simulink model "Vehicle_Dynamic_Simulator"  (R2021b)
settings: Solver=VariableStepAuto  StartTime=0.0  StopTime=200  RelTol=1e-3
undefined symbols (not defined in the file): Path
libraries: Solver_SF x2, mpclib x1, sldrtlib x1
(part 1 of 2)
settings Model: Creator=li.ang  LastModifiedBy=li.ang
settings SFSimCC: SimTargetLang=C++
settings ConfigComp: PLC_TargetIDE=codesys23  PLC_MultiTBSigbuilderTimeRange=off  PLC_InlineEnumCastFunction=off

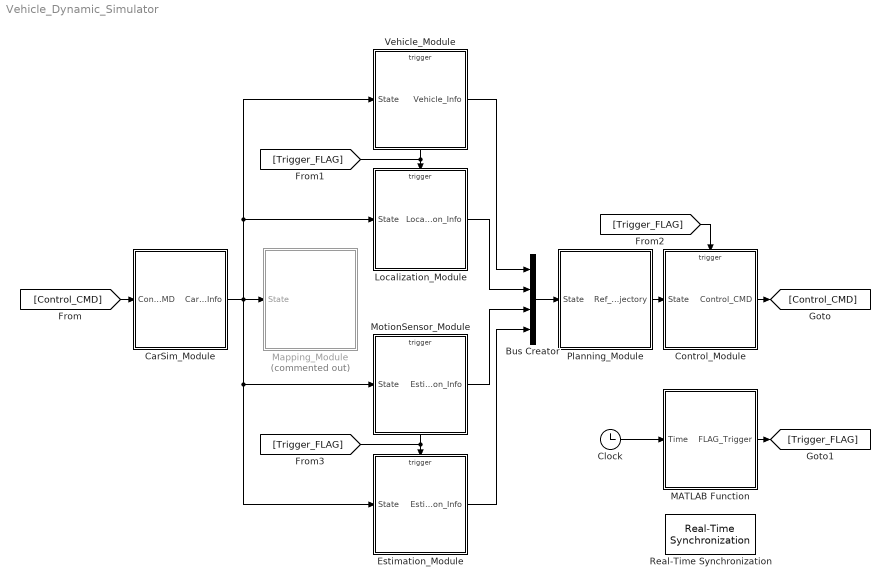
== system Vehicle_Dynamic_Simulator ==
  Bus Creator : BusCreator  Inputs=4
  CarSim_Module : Subsystem  mask{LonFlag=on, LatFlag=on}
      mask prompts: LonFlag "use custom lon controller"; LatFlag "use custom lat controller"
      mask Display: image('TruckSim.png'); % 使用工具条上的 "编辑图像" 进行更改。
  Clock : Clock
  Control_Module : Subsystem
  Estimation_Module : Subsystem  mask{VehicleFlag=Truck_106_Daimler_Auman, ModelFlag=Static 2DOF Vehicle Model}
      mask prompts: VehicleFlag "Select Test Vehicle"; ModelFlag "Model Type"
      mask TypeOptions VehicleFlag: Truck_106_Daimler_Auman
      mask TypeOptions ModelFlag: Static 2DOF Vehicle Model | Static 2DOF Error Model | Dynamic 2DOF Vehicle Model | Dynamic 2DOF Error Model
      mask Display: addpath('Pictures');
  Localization_Module : Subsystem  mask{FLAGS_choose_path=Test: Step Curvature Response: 10m Radius, FLAGS_enable_preview=on, FLAGS_preview_window=0}
      mask prompts: FLAGS_choose_path "Select Path"; FLAGS_enable_preview "Enable Preview"; FLAGS_preview_window "Input Preview Window"
      mask init:
      | % Add Search Path
      | addpath('Scenarios');
      | addpath('Scenarios\Scenario_Test_Flat_Pad');
      | 
      | % Test Road Selector
      | switch FLAGS_choose_path
      |     case 1
      |         load('Path_Curvature_Step_Response_8m_Radius.mat');
      |     case 2
      |         load('Path_Curvature_Step_Response_10m_Radius.mat');
      |     case 3
      |         load('Path_Curvature_Step_Response_16m_Radius.mat');
      |     case 4
      |         load('Path_Curvature_Step_Response_20m_Radius.mat');
      |     case 5
      |         load('Path_Curvature_Step_Response_40m_Radius.mat');
      |     case 6
      |         load('Path_Curvature_Step_Response_50m_Radius.mat');
      |     case 7
      |         load('Path_Curvature_Step_Response_80m_Radius.mat');
      |     case 8
      |         load('Path_Curvature_Step_Response_100m_Radius.mat');
      | 
      | %     case 2
      | %         load('MCity_M_Loop.mat')
      | % 
      | %     case 3      % Road: Course2D
      | %         load('Path_HandlingCourse.mat');
      | % 
      | %     case 8      % Road: Course3D
      | %         Path = load('Course3D.mat');
      | %         Index      = Path.Road.Index
      | %         Station    = Path.Road.S;
      | %         X_Global   = Path.Road.X;
      | %         Y_Global   = Path.Road.Y;
      | %         Theta      = Path.Road.Theta;
      | %         Kappa      = Path.Road.Kappa; 
      |         
      | %     case 1      % Step Curvature: Kappa = 0.01
      | %         Centerline = load('Step_Kappa_0.01.mat');
      | %         Index      = Centerline.Road.Index
      | %         Station    = Centerline.Road.S;
      | %         X_Global   = Centerline.Road.X;
      | %         Y_Global   = Centerline.Road.Y;
      | %         Theta      = Centerline.Road.Theta;
      | %         Kappa      = Centerline.Road.Kappa;
      | %     case 2      % Step Curvature: Kappa = 0.02
      | %         Centerline = load('Step_Kappa_0.02.mat');
      | %         Index      = Centerline.Road.Index
      | %         Station    = Centerline.Road.S;
      | %         X_Global   = Centerline.Road.X;
      | %         Y_Global   = Centerline.Road.Y;
      | %         Theta      = Centerline.Road.Theta;
      | %         Kappa      = Centerline.Road.Kappa;  
      | %     case 3      % Step Curvature: Kappa = 0.05
      | %         Centerline = load('Step_Kappa_0.05.mat');
      | %         Index      = Centerline.Road.Index
      | %         Station    = Centerline.Road.S;
      | %         X_Global   = Centerline.Road.X;
      | %         Y_Global   = Centerline.Road.Y;
      | %         Theta      = Centerline.Road.Theta;
      | %         Kappa      = Centerline.Road.Kappa;
      | %     case 4      % Ramp Curvature: dKappa = 0.01
      | %         Centerline = load('Ramp_dKappa_0.01.mat');
      | %         Index      = Centerline.Road.Index
      | %         Station    = Centerline.Road.S;
      | %         X_Global   = Centerline.Road.X;
      | %         Y_Global   = Centerline.Road.Y;
      | %         Theta      = Centerline.Road.Theta;
      | %         Kappa      = Centerline.Road.Kappa;
      | %     case 5      % Road: uTurn
      | %         Centerline = load('uTurn.mat');
      | %         Index      = Centerline.Road.Index
      | %         Station    = Centerline.Road.S;
      | %         X_Global   = Centerline.Road.X;
      | %         Y_Global   = Centerline.Road.Y;
      | %         Theta      = Centerline.Road.Theta;
      | %         Kappa      = Centerline.Road.Kappa;
      | %     case 6      % Road: Highway
      | %         Centerline = load('Highway.mat');
      | %         Index      = Centerline.Road.Index
      | %         Station    = Centerline.Road.S;
      | %         X_Global   = Centerline.Road.X;
      | %         Y_Global   = Centerline.Road.Y;
      | %         Theta      = Centerline.Road.Theta;
      | %         Kappa      = Centerline.Road.Kappa;
      | end
      mask TypeOptions FLAGS_choose_path: Test: Step Curvature Response: 8m Radius | Test: Step Curvature Response: 10m Radius | Test: Step Curvature Response: 16m Radius | Test: Step Curvature Response: 20m Radius | Test: Step Curvature Response: 40m Radius | Test: Step Curvature Response: 50m Radius | Test: Step Curvature Response: 80m Radius | Test: Step Curvature Response: 100m Radius
      mask Display:
      | addpath('Pictures');
      | image('Road.png');
  MATLAB Function : MATLAB Function  TreatAsAtomicUnit=on
  Mapping_Module : Subsystem  Commented=on
  MotionSensor_Module : Subsystem  mask{VehicleFlag=Truck_106_Daimler_Auman, ModelFlag=Static 2DOF Vehicle Model}
      mask prompts: VehicleFlag "Select Test Vehicle"; ModelFlag "Model Type"
      mask TypeOptions VehicleFlag: Truck_106_Daimler_Auman
      mask TypeOptions ModelFlag: Static 2DOF Vehicle Model | Static 2DOF Error Model | Dynamic 2DOF Vehicle Model | Dynamic 2DOF Error Model
      mask Display: addpath('Pictures');
  Planning_Module : Subsystem
  Real-Time Synchronization : sldrtlib/Real-Time Synchronization  SampleTime=0.1  MaxMissedTicks=10  ShowMissedTicks=off  YieldWhenWaiting=off
  Vehicle_Module : Subsystem  mask{VehicleFlag=Truck_106_Daimler_Auman, ModelFlag=Static 2DOF Vehicle Model}
      mask prompts: VehicleFlag "Select Test Vehicle"; ModelFlag "Model Type"
      mask init:
      | % Add Search Path
      | addpath('Vehicles');
      | 
      | % Test Vehicle Selector
      | % switch VehicleFlag
      | %     case 1
      | %         Vehicle         = load('Truck_106_Daimler_Auman.mat').Vehicle;
      | %         TotalMass       = Vehicle.TotalMass;
      | %         TotalInertia    = Vehicle.TotalInertia;
      | %         TyreStiffness   = Vehicle.AxleStiffness;
      | %         AxlePosition    = Vehicle.AxlePosition;
      | %     case 2
      | %     case 3
      | %     case 4
      | %         Vehicle         = load('Truck_106_Daimler_Auman.mat').Vehicle;
      | %         TotalMass       = Vehicle.TotalMass;
      | %         TotalInertia    = Vehicle.TotalInertia;
      | %         TyreStiffness   = Vehicle.AxleStiffness;
      | %         AxlePosition    = Vehicle.AxlePosition;
      | %         ...
      | % end
      mask TypeOptions VehicleFlag: Truck_106_Daimler_Auman
      mask TypeOptions ModelFlag: Static 2DOF Vehicle Model | Static 2DOF Error Model | Dynamic 2DOF Vehicle Model | Dynamic 2DOF Error Model
      mask Display:
      | addpath('Pictures');
      | image('Vehicle_Module.png');
  wires:
  CarSim_Module/1(CarSim_Info) -> Mapping_Module/1(State), Estimation_Module/1(State), MotionSensor_Module/1(State), Vehicle_Module/1(State), Localization_Module/1(State)
  Control_Module/1(Control_CMD) -> [Control_CMD]
  Bus Creator/1 -> Planning_Module/1(State)
  Planning_Module/1(Ref_Trajectory) -> Control_Module/1(State)
  MATLAB Function/1(FLAG_Trigger) -> [Trigger_FLAG]
  Clock/1 -> MATLAB Function/1(Time)
  [Trigger_FLAG] -> Localization_Module/Trigger, Vehicle_Module/Trigger
  [Trigger_FLAG] -> Control_Module/Trigger
  [Trigger_FLAG] -> Estimation_Module/Trigger, MotionSensor_Module/Trigger
  [Control_CMD] -> CarSim_Module/1(Control_CMD)
  Vehicle_Module/1(Vehicle_Info) -> Bus Creator/1
  Localization_Module/1(Localization_Info) -> Bus Creator/2
  MotionSensor_Module/1(Estimation_Info) -> Bus Creator/3
  Estimation_Module/1(Estimation_Info) -> Bus Creator/4

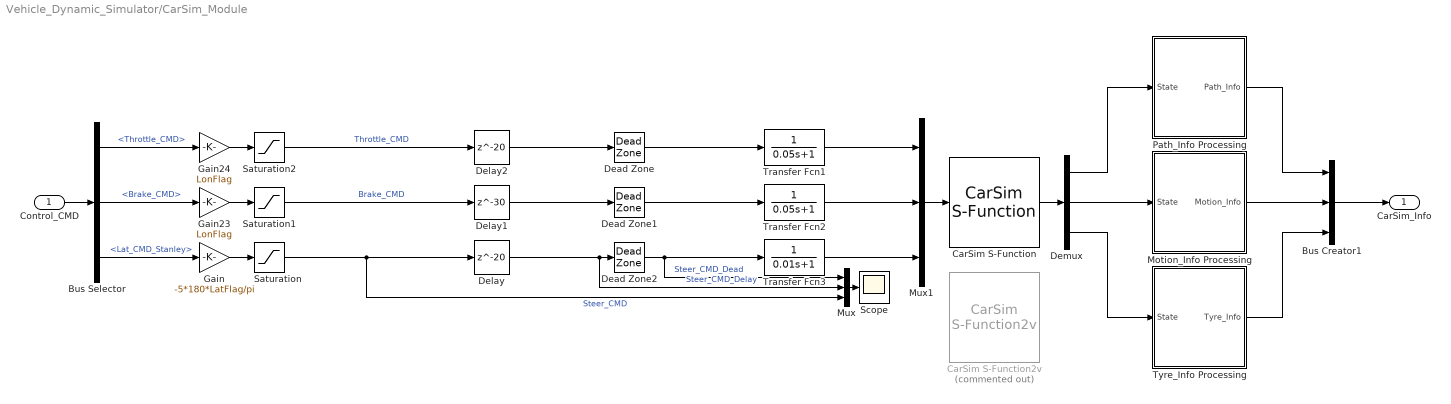
== system Vehicle_Dynamic_Simulator/CarSim_Module ==
  Control_CMD : Inport
  Bus Creator1 : BusCreator  Inputs=3
  Bus Selector : BusSelector  OutputSignals=Lon_CMD.Throttle_CMD,Lon_CMD.Brake_CMD,Lat_CMD.Lat_CMD_Stanley
  CarSim S-Function : Solver_SF/CarSim S-Function  Priority=1  SIMFILE=simfile.sim
  CarSim S-Function2v : Solver_SF/CarSim S-Function2v  Priority=1  Commented=on  SIMFILE=CarSimfile.sim
      settings: SourceProductName=CarSim S-Function
  Dead Zone : DeadZone  LowerValue=0  UpperValue=0.05  SaturateOnIntegerOverflow=on
  Dead Zone1 : DeadZone  LowerValue=0  UpperValue=0.05  SaturateOnIntegerOverflow=on
  Dead Zone2 : DeadZone  LowerValue=-1  UpperValue=1  SaturateOnIntegerOverflow=on
  Delay : Delay  DelayLength=20
  Delay1 : Delay  DelayLength=30  SampleTime=0.01
  Delay2 : Delay  DelayLength=20  SampleTime=0.01
  Demux : Demux  Outputs=[14, 20, 44]
  Gain : Gain  Gain=-5*180*LatFlag/pi
  Gain23 : Gain  Gain=LonFlag
  Gain24 : Gain  Gain=LonFlag
  Motion_Info Processing : Subsystem
  Mux : Mux  Inputs=3
  Mux1 : Mux  Inputs=3
  Path_Info Processing : Subsystem
  Saturation : Saturate  UpperLimit=+540  LowerLimit=-540
  Saturation1 : Saturate  UpperLimit=+1000  LowerLimit=-1000
  Saturation2 : Saturate  UpperLimit=+1000  LowerLimit=-1000
  Scope : Scope
  Transfer Fcn1 : TransferFcn  Denominator=[0.05 1]
  Transfer Fcn2 : TransferFcn  Denominator=[0.05 1]
  Transfer Fcn3 : TransferFcn  Denominator=[0.01 1]
  Tyre_Info Processing : Subsystem
  CarSim_Info : Outport
  wires:
  Bus Creator1/1 -> CarSim_Info/1
  Mux1/1 -> CarSim S-Function/1
  Demux/1 -> Path_Info Processing/1(State)
  CarSim S-Function/1 -> Demux/1
  Demux/2 -> Motion_Info Processing/1(State)
  Demux/3 -> Tyre_Info Processing/1(State)
  Motion_Info Processing/1(Motion_Info) -> Bus Creator1/2
  Path_Info Processing/1(Path_Info) -> Bus Creator1/1
  Tyre_Info Processing/1(Tyre_Info) -> Bus Creator1/3
  Saturation/1 -> Mux/3, Delay/1  "Steer_CMD"
  Dead Zone/1 -> Transfer Fcn1/1
  Mux/1 -> Scope/1
  Dead Zone1/1 -> Transfer Fcn2/1
  Delay/1 -> Mux/2, Dead Zone2/1  "Steer_CMD_Delay"
  Gain23/1 -> Saturation1/1
  Control_CMD/1 -> Bus Selector/1
  Delay2/1 -> Dead Zone/1
  Gain24/1 -> Saturation2/1
  Saturation2/1 -> Delay2/1  "Throttle_CMD"
  Dead Zone2/1 -> Mux/1, Transfer Fcn3/1  "Steer_CMD_Dead"
  Delay1/1 -> Dead Zone1/1
  Saturation1/1 -> Delay1/1  "Brake_CMD"
  Gain/1 -> Saturation/1
  Bus Selector/1 -> Gain24/1  "<Throttle_CMD>"
  Bus Selector/2 -> Gain23/1  "<Brake_CMD>"
  Bus Selector/3 -> Gain/1  "<Lat_CMD_Stanley>"
  Transfer Fcn2/1 -> Mux1/2
  Transfer Fcn1/1 -> Mux1/1
  Transfer Fcn3/1 -> Mux1/3

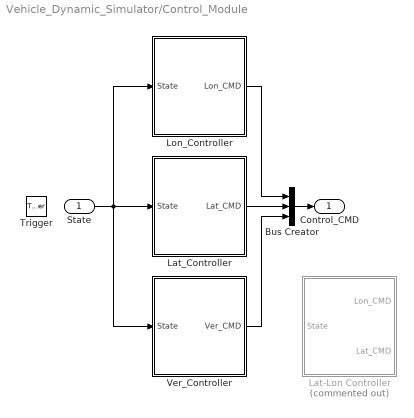
== system Vehicle_Dynamic_Simulator/Control_Module ==
  State : Inport
  Trigger : TriggerPort  VariantControl=(inherit)  PortDimensions=1
  Bus Creator : BusCreator  Inputs=3
  Lat-Lon Controller : Subsystem  Commented=on
  Lat_Controller : Subsystem
  Lon_Controller : Subsystem
  Ver_Controller : Subsystem
  Control_CMD : Outport
  wires:
  Bus Creator/1 -> Control_CMD/1
  Lon_Controller/1(Lon_CMD) -> Bus Creator/1
  State/1 -> Ver_Controller/1(State), Lat_Controller/1(State), Lon_Controller/1(State)
  Lat_Controller/1(Lat_CMD) -> Bus Creator/2
  Ver_Controller/1(Ver_CMD) -> Bus Creator/3

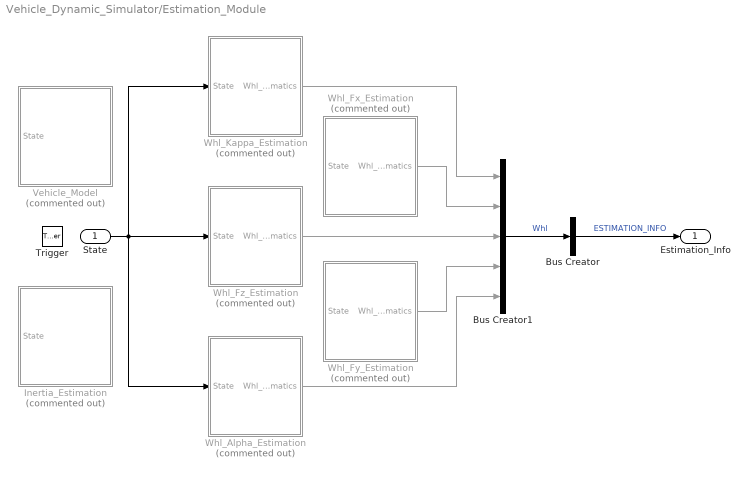
== system Vehicle_Dynamic_Simulator/Estimation_Module ==
  State : Inport
  Trigger : TriggerPort  VariantControl=(inherit)  PortDimensions=1
  Bus Creator : BusCreator  Inputs=1
  Bus Creator1 : BusCreator  Inputs=5
  Inertia_Estimation : Subsystem  Commented=on
  Vehicle_Model : Subsystem  Commented=on
  Whl_Alpha_Estimation : Subsystem  Commented=on
  Whl_Fx_Estimation : Subsystem  Commented=on
  Whl_Fy_Estimation : Subsystem  Commented=on
  Whl_Fz_Estimation : Subsystem  Commented=on
  Whl_Kappa_Estimation : Subsystem  Commented=on
  Estimation_Info : Outport
  wires:
  State/1 -> Whl_Fz_Estimation/1(State), Whl_Alpha_Estimation/1(State), Whl_Kappa_Estimation/1(State)
  Bus Creator/1 -> Estimation_Info/1  "ESTIMATION_INFO"
  Whl_Kappa_Estimation/1(Whl_Kinematics) -> Bus Creator1/1
  Bus Creator1/1 -> Bus Creator/1  "Whl"
  Whl_Fz_Estimation/1(Whl_Kinematics) -> Bus Creator1/3
  Whl_Fx_Estimation/1(Whl_Kinematics) -> Bus Creator1/2
  Whl_Fy_Estimation/1(Whl_Kinematics) -> Bus Creator1/4
  Whl_Alpha_Estimation/1(Whl_Kinematics) -> Bus Creator1/5

== system Vehicle_Dynamic_Simulator/Localization_Module ==
  State : Inport
  Trigger : TriggerPort  VariantControl=(inherit)  PortDimensions=1
  Bus Creator : BusCreator  Inputs=3
  Error_Calculation : Subsystem
  Geo_Calculation : Subsystem
  Prev_Calculation : Subsystem
  Localization_Info : Outport
  wires:
  State/1 -> Geo_Calculation/1(State), Prev_Calculation/1(State), Error_Calculation/1(State)
  Bus Creator/1 -> Localization_Info/1  "LOCALIZATION_INFO"
  Error_Calculation/1(Path_Error_Info) -> Bus Creator/1
  Prev_Calculation/1(Path_Prev_Info) -> Bus Creator/3
  Geo_Calculation/1(Path_Error_Info) -> Bus Creator/2

== system Vehicle_Dynamic_Simulator/Mapping_Module ==
  State : Inport
  Bus Selector : BusSelector  OutputSignals=PATH_INFO.Path_S_Ref,PATH_INFO.Path_X_Ref,PATH_INFO.Path_Y_Ref,PATH_INFO.Path_Kappa_Ref
  Scope : Scope  NumInputPorts=4
  To Workspace : ToWorkspace  VariableName=S  SaveFormat=Timeseries  SampleTime=0.02
  To Workspace1 : ToWorkspace  VariableName=X  SaveFormat=Timeseries  SampleTime=0.02
  To Workspace2 : ToWorkspace  VariableName=Y  SaveFormat=Timeseries  SampleTime=0.02
  To Workspace3 : ToWorkspace  VariableName=Kappa  SaveFormat=Timeseries  SampleTime=0.02
  wires:
  State/1 -> Bus Selector/1
  Bus Selector/1 -> To Workspace/1, Scope/1  "<Path_S_Ref>"
  Bus Selector/2 -> To Workspace1/1, Scope/2  "<Path_X_Ref>"
  Bus Selector/3 -> To Workspace2/1, Scope/3  "<Path_Y_Ref>"
  Bus Selector/4 -> Scope/4, To Workspace3/1  "<Path_Kappa_Ref>"

== system Vehicle_Dynamic_Simulator/MotionSensor_Module ==
  State : Inport
  Trigger : TriggerPort  VariantControl=(inherit)  PortDimensions=1
  Bus Selector : BusSelector  OutputSignals=MOTION_INFO
  Estimation_Info : Outport
  wires:
  Bus Selector/1 -> Estimation_Info/1  "<MOTION_INFO>"
  State/1 -> Bus Selector/1

== system Vehicle_Dynamic_Simulator/Planning_Module ==
  State : Inport
  Ref_Trajectory : Outport
  wires:
  State/1 -> Ref_Trajectory/1

== system Vehicle_Dynamic_Simulator/Vehicle_Module ==
  State : Inport
  Trigger : TriggerPort  VariantControl=(inherit)  PortDimensions=1
  Vehicle_Info : Outport
  wires:
  State/1 -> Vehicle_Info/1  "VEHICLE_INFO"

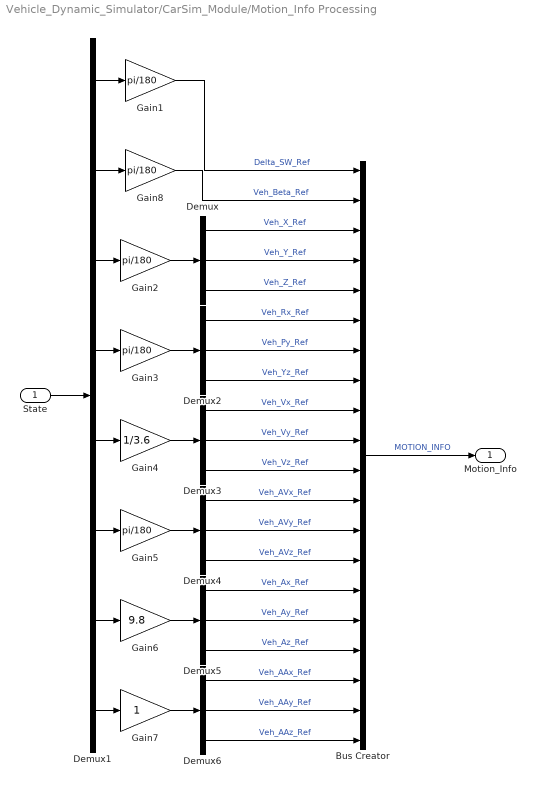
== system Vehicle_Dynamic_Simulator/CarSim_Module/Motion_Info Processing ==
  State : Inport
  Bus Creator : BusCreator  Inputs=20
  Demux{,2..6} (6 alike) : Demux  Outputs=3
  Demux1 : Demux  Outputs=[1, 1, 3, 3, 3, 3, 3, 3]
  Gain{1..3,5,8} (5 alike) : Gain  Gain=pi/180
  Gain4 : Gain  Gain=1/3.6
  Gain6 : Gain  Gain=9.8
  Gain7 : Gain
  Motion_Info : Outport
  wires:
  State/1 -> Demux1/1
  Bus Creator/1 -> Motion_Info/1  "MOTION_INFO"
  Demux1/1 -> Gain1/1
  Gain1/1 -> Bus Creator/1  "Delta_SW_Ref"
  Demux1/6 -> Gain5/1
  Demux5/1 -> Bus Creator/15  "Veh_Ax_Ref"
  Demux4/1 -> Bus Creator/12  "Veh_AVx_Ref"
  Demux1/5 -> Gain4/1
  Demux5/2 -> Bus Creator/16  "Veh_Ay_Ref"
  Demux4/2 -> Bus Creator/13  "Veh_AVy_Ref"
  Demux3/2 -> Bus Creator/10  "Veh_Vy_Ref"
  Demux3/3 -> Bus Creator/11  "Veh_Vz_Ref"
  Gain7/1 -> Demux6/1
  Demux1/8 -> Gain7/1
  Demux4/3 -> Bus Creator/14  "Veh_AVz_Ref"
  Demux6/2 -> Bus Creator/19  "Veh_AAy_Ref"
  Demux1/7 -> Gain6/1
  Demux6/1 -> Bus Creator/18  "Veh_AAx_Ref"
  Gain5/1 -> Demux4/1
  Demux5/3 -> Bus Creator/17  "Veh_Az_Ref"
  Demux3/1 -> Bus Creator/9  "Veh_Vx_Ref"
  Gain4/1 -> Demux3/1
  Gain6/1 -> Demux5/1
  Demux6/3 -> Bus Creator/20  "Veh_AAz_Ref"
  Demux/3 -> Bus Creator/5  "Veh_Z_Ref"
  Demux1/4 -> Gain3/1
  Gain3/1 -> Demux2/1
  Demux2/2 -> Bus Creator/7  "Veh_Py_Ref"
  Demux/2 -> Bus Creator/4  "Veh_Y_Ref"
  Demux1/3 -> Gain2/1
  Gain2/1 -> Demux/1
  Demux2/3 -> Bus Creator/8  "Veh_Yz_Ref"
  Demux/1 -> Bus Creator/3  "Veh_X_Ref"
  Demux2/1 -> Bus Creator/6  "Veh_Rx_Ref"
  Demux1/2 -> Gain8/1
  Gain8/1 -> Bus Creator/2  "Veh_Beta_Ref"

== system Vehicle_Dynamic_Simulator/CarSim_Module/Path_Info Processing ==
  State : Inport
  Bus Creator2 : BusCreator  Inputs=7
  Demux3 : Demux  Outputs=[1, 1, 1, 1, 1, 4, 5]
  Path_Info : Outport
  wires:
  Demux3/5 -> Bus Creator2/5  "Path_Kappa_Ref"
  Bus Creator2/1 -> Path_Info/1  "PATH_INFO"
  Demux3/3 -> Bus Creator2/3  "Path_X_Ref"
  Demux3/6 -> Bus Creator2/6  "Veh_L_drv_Ref"
  Demux3/1 -> Bus Creator2/1  "Path_S_Ref"
  Demux3/2 -> Bus Creator2/2  "Path_L_Ref"
  Demux3/4 -> Bus Creator2/4  "Path_Y_Ref"
  State/1 -> Demux3/1
  Demux3/7 -> Bus Creator2/7  "Veh_A_drv_Ref"

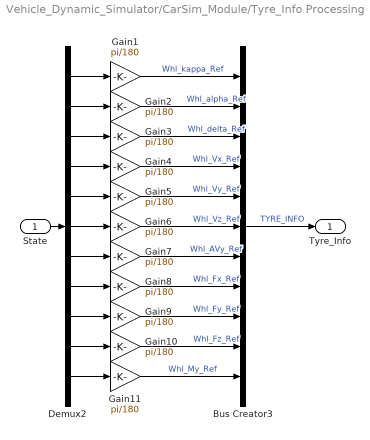
== system Vehicle_Dynamic_Simulator/CarSim_Module/Tyre_Info Processing ==
  State : Inport
  Bus Creator3 : BusCreator  Inputs=11
  Demux2 : Demux  Outputs=[4, 4, 4, 4, 4, 4, 4, 4, 4, 4, 4]
  Gain{1..11} (11 alike) : Gain  Gain=pi/180
  Tyre_Info : Outport
  wires:
  Demux2/5 -> Gain5/1
  Demux2/6 -> Gain6/1
  Gain7/1 -> Bus Creator3/7  "Whl_AVy_Ref"
  Gain5/1 -> Bus Creator3/5  "Whl_Vy_Ref"
  Demux2/7 -> Gain7/1
  Gain4/1 -> Bus Creator3/4  "Whl_Vx_Ref"
  Demux2/4 -> Gain4/1
  Demux2/2 -> Gain2/1
  Demux2/3 -> Gain3/1
  Gain6/1 -> Bus Creator3/6  "Whl_Vz_Ref"
  Gain3/1 -> Bus Creator3/3  "Whl_delta_Ref"
  Gain2/1 -> Bus Creator3/2  "Whl_alpha_Ref"
  State/1 -> Demux2/1
  Bus Creator3/1 -> Tyre_Info/1  "TYRE_INFO"
  Demux2/11 -> Gain11/1
  Gain11/1 -> Bus Creator3/11  "Whl_My_Ref"
  Gain10/1 -> Bus Creator3/10  "Whl_Fz_Ref"
  Gain9/1 -> Bus Creator3/9  "Whl_Fy_Ref"
  Gain8/1 -> Bus Creator3/8  "Whl_Fx_Ref"
  Demux2/8 -> Gain8/1
  Demux2/9 -> Gain9/1
  Demux2/10 -> Gain10/1
  Demux2/1 -> Gain1/1
  Gain1/1 -> Bus Creator3/1  "Whl_kappa_Ref"

== system Vehicle_Dynamic_Simulator/Control_Module/Lat-Lon Controller ==
  State : Inport
  Bus Selector : BusSelector  OutputSignals=LOCALIZATION_INFO.PATH_ERROR_INFO,LOCALIZATION_INFO.PATH_GEO_INFO,MOTION_INFO.Veh_Beta_Ref,MOTION_INFO.Veh_Vx_Ref,MOTION_INFO.Veh_Vy_Ref
  MATLAB Function2 : MATLAB Function  TreatAsAtomicUnit=on
  Lon_CMD : Outport
  Lat_CMD : Outport  Port=2
  wires:
  State/1 -> Bus Selector/1

== system Vehicle_Dynamic_Simulator/Control_Module/Lat_Controller ==
  State : Inport
  Bus Creator : BusCreator  Inputs=3
  Offline_LQR_Controller : Subsystem  Commented=on
  Offline_OPC_Controller : Subsystem  Commented=on
  Online_MPC_Controller : Subsystem  Commented=on
  Stanley_Controller : Subsystem
  Lat_CMD : Outport
  wires:
  State/1 -> Stanley_Controller/1(State), Offline_OPC_Controller/1(State), Online_MPC_Controller/1(State), Offline_LQR_Controller/1(State)
  Bus Creator/1 -> Lat_CMD/1  "Lat_CMD"
  Stanley_Controller/1(Lat_CMD) -> Bus Creator/1  "Lat_CMD_Stanley"
  Offline_LQR_Controller/1(Lat_CMD) -> Bus Creator/2  "Lat_CMD_LQR"
  Offline_OPC_Controller/1(Lat_CMD) -> Bus Creator/3  "Lat_CMD_OPC"

== system Vehicle_Dynamic_Simulator/Control_Module/Lon_Controller ==
  State : Inport
  Bus Creator : BusCreator  Inputs=2
  Constant : Constant  Value=0
  Constant1 : Constant  Value=0
  Terminator : Terminator
  Lon_CMD : Outport
  wires:
  Bus Creator/1 -> Lon_CMD/1  "Lon_CMD"
  Constant/1 -> Bus Creator/1  "Throttle_CMD"
  Constant1/1 -> Bus Creator/2  "Brake_CMD"
  State/1 -> Terminator/1

== system Vehicle_Dynamic_Simulator/Control_Module/Ver_Controller ==
  State : Inport
  Bus Creator : BusCreator  Inputs=3
  Ver_CMD : Outport
  wires:
  Bus Creator/1 -> Ver_CMD/1  "Ver_CMD"

== system Vehicle_Dynamic_Simulator/Estimation_Module/Inertia_Estimation ==
  State : Inport

== system Vehicle_Dynamic_Simulator/Estimation_Module/Vehicle_Model ==
  State : Inport
  7DOF_Model : Subsystem
      mask init:
      | % Add Search Path
      | addpath('Tyre');
      | 
      | % Test Road Selector
      | Tyre = load('Tyre_265_70_R17');
      | Alpha = Tyre.Alpha;
      | Kappa = Tyre.Kappa;
      | 
      | Fx = Tyre.Fx;
      | Fy = Tyre.Fy;
      | Fz = Tyre.Fz;
  wires:
  State/1 -> 7DOF_Model/1(State)

== system Vehicle_Dynamic_Simulator/Estimation_Module/Whl_Alpha_Estimation ==
  State : Inport
  Bus Selector : BusSelector  OutputSignals=MOTION_INFO.Delta_SW_Ref,MOTION_INFO.Veh_Vx_Ref,MOTION_INFO.Veh_Vy_Ref,MOTION_INFO.Veh_AVz_Ref,TYRE_INFO.Whl_AVy_Ref
  Wheel_Kinematics_Estimation : MATLAB Function  TreatAsAtomicUnit=on
  Whl_Kinematics : Outport
  wires:
  Bus Selector/5 -> Wheel_Kinematics_Estimation/5(Whl_AVy_Ref)  "<Whl_AVy_Ref>"
  Bus Selector/4 -> Wheel_Kinematics_Estimation/4(Veh_AVz_Ref)  "<Veh_AVz_Ref>"
  Bus Selector/1 -> Wheel_Kinematics_Estimation/1(Delta_SW_Ref)  "<Delta_SW_Ref>"
  Bus Selector/2 -> Wheel_Kinematics_Estimation/2(Veh_Vx_Ref)  "<Veh_Vx_Ref>"
  Bus Selector/3 -> Wheel_Kinematics_Estimation/3(Veh_Vy_Ref)  "<Veh_Vy_Ref>"
  State/1 -> Bus Selector/1
  Wheel_Kinematics_Estimation/2(Whl_Alpha) -> Whl_Kinematics/1  "Whl_Alpha_Est"

== system Vehicle_Dynamic_Simulator/Estimation_Module/Whl_Fx_Estimation ==
  State : Inport
  Bus Selector : BusSelector  OutputSignals=MOTION_INFO.Delta_SW_Ref,MOTION_INFO.Veh_Vx_Ref,MOTION_INFO.Veh_Vy_Ref,MOTION_INFO.Veh_AVz_Ref,TYRE_INFO.Whl_AVy_Ref
  Wheel_Kinematics_Estimation : MATLAB Function  TreatAsAtomicUnit=on
  Whl_Kinematics : Outport
  wires:
  Bus Selector/5 -> Wheel_Kinematics_Estimation/5(Whl_AVy_Ref)  "<Whl_AVy_Ref>"
  Bus Selector/4 -> Wheel_Kinematics_Estimation/4(Veh_AVz_Ref)  "<Veh_AVz_Ref>"
  Bus Selector/1 -> Wheel_Kinematics_Estimation/1(Delta_SW_Ref)  "<Delta_SW_Ref>"
  Bus Selector/2 -> Wheel_Kinematics_Estimation/2(Veh_Vx_Ref)  "<Veh_Vx_Ref>"
  Bus Selector/3 -> Wheel_Kinematics_Estimation/3(Veh_Vy_Ref)  "<Veh_Vy_Ref>"
  State/1 -> Bus Selector/1
  Wheel_Kinematics_Estimation/1(Whl_Kappa) -> Whl_Kinematics/1  "Whl_Fx_Est"

== system Vehicle_Dynamic_Simulator/Estimation_Module/Whl_Fy_Estimation ==
  State : Inport
  Bus Selector : BusSelector  OutputSignals=MOTION_INFO.Delta_SW_Ref,MOTION_INFO.Veh_Vx_Ref,MOTION_INFO.Veh_Vy_Ref,MOTION_INFO.Veh_AVz_Ref,TYRE_INFO.Whl_AVy_Ref
  Wheel_Kinematics_Estimation : MATLAB Function  TreatAsAtomicUnit=on
  Whl_Kinematics : Outport
  wires:
  State/1 -> Bus Selector/1
  Bus Selector/3 -> Wheel_Kinematics_Estimation/3(Veh_Vy_Ref)  "<Veh_Vy_Ref>"
  Bus Selector/2 -> Wheel_Kinematics_Estimation/2(Veh_Vx_Ref)  "<Veh_Vx_Ref>"
  Bus Selector/1 -> Wheel_Kinematics_Estimation/1(Delta_SW_Ref)  "<Delta_SW_Ref>"
  Bus Selector/4 -> Wheel_Kinematics_Estimation/4(Veh_AVz_Ref)  "<Veh_AVz_Ref>"
  Bus Selector/5 -> Wheel_Kinematics_Estimation/5(Whl_AVy_Ref)  "<Whl_AVy_Ref>"
  Wheel_Kinematics_Estimation/1(Whl_Kappa) -> Whl_Kinematics/1  "Whl_Fy_Est"

== system Vehicle_Dynamic_Simulator/Estimation_Module/Whl_Fz_Estimation ==
  State : Inport
  Bus Selector : BusSelector  OutputSignals=MOTION_INFO.Delta_SW_Ref,MOTION_INFO.Veh_Vx_Ref,MOTION_INFO.Veh_Vy_Ref,MOTION_INFO.Veh_AVz_Ref,TYRE_INFO.Whl_AVy_Ref
  Wheel_Kinematics_Estimation : MATLAB Function  TreatAsAtomicUnit=on
  Whl_Kinematics : Outport
  wires:
  State/1 -> Bus Selector/1
  Bus Selector/3 -> Wheel_Kinematics_Estimation/3(Veh_Vy_Ref)  "<Veh_Vy_Ref>"
  Bus Selector/2 -> Wheel_Kinematics_Estimation/2(Veh_Vx_Ref)  "<Veh_Vx_Ref>"
  Bus Selector/1 -> Wheel_Kinematics_Estimation/1(Delta_SW_Ref)  "<Delta_SW_Ref>"
  Bus Selector/4 -> Wheel_Kinematics_Estimation/4(Veh_AVz_Ref)  "<Veh_AVz_Ref>"
  Bus Selector/5 -> Wheel_Kinematics_Estimation/5(Whl_AVy_Ref)  "<Whl_AVy_Ref>"
  ? -> Whl_Kinematics/1  "Whl_Fz_Est"

== system Vehicle_Dynamic_Simulator/Estimation_Module/Whl_Kappa_Estimation ==
  State : Inport
  Bus Selector : BusSelector  OutputSignals=MOTION_INFO.Delta_SW_Ref,MOTION_INFO.Veh_Vx_Ref,MOTION_INFO.Veh_Vy_Ref,MOTION_INFO.Veh_AVz_Ref,TYRE_INFO.Whl_AVy_Ref
  Wheel_Kinematics_Estimation : MATLAB Function  TreatAsAtomicUnit=on
  Whl_Kinematics : Outport
  wires:
  State/1 -> Bus Selector/1
  Bus Selector/3 -> Wheel_Kinematics_Estimation/3(Veh_Vy_Ref)  "<Veh_Vy_Ref>"
  Bus Selector/2 -> Wheel_Kinematics_Estimation/2(Veh_Vx_Ref)  "<Veh_Vx_Ref>"
  Bus Selector/1 -> Wheel_Kinematics_Estimation/1(Delta_SW_Ref)  "<Delta_SW_Ref>"
  Bus Selector/4 -> Wheel_Kinematics_Estimation/4(Veh_AVz_Ref)  "<Veh_AVz_Ref>"
  Bus Selector/5 -> Wheel_Kinematics_Estimation/5(Whl_AVy_Ref)  "<Whl_AVy_Ref>"
  Wheel_Kinematics_Estimation/1(Whl_Kappa) -> Whl_Kinematics/1  "Whl_Kappa_Est"

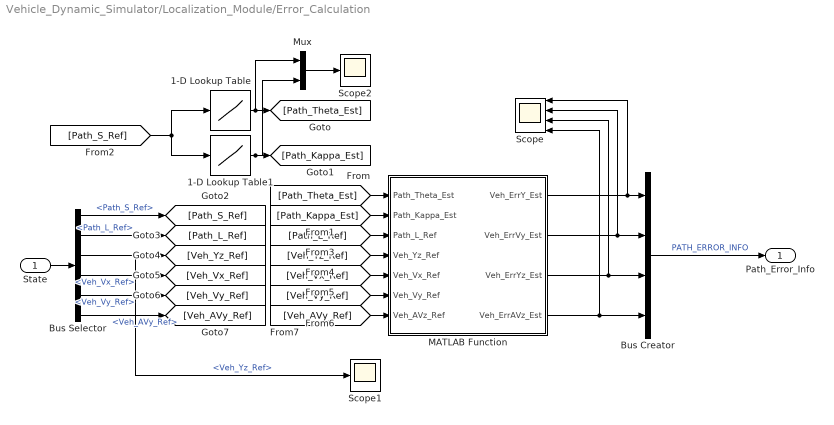
== system Vehicle_Dynamic_Simulator/Localization_Module/Error_Calculation ==
  State : Inport
  1-D Lookup Table : Lookup_n-D  NumberOfTableDimensions=1  BreakpointsForDimension1=Path.S  Table=Path.Theta  InternalRulePriority=Speed  RndMeth=Simplest  InputSameDT=on
  1-D Lookup Table1 : Lookup_n-D  NumberOfTableDimensions=1  BreakpointsForDimension1=Path.S  Table=Path.Kappa  InternalRulePriority=Speed  RndMeth=Simplest  InputSameDT=on
  Bus Creator : BusCreator  Inputs=4
  Bus Selector : BusSelector  OutputSignals=PATH_INFO.Path_S_Ref,PATH_INFO.Path_L_Ref,MOTION_INFO.Veh_Yz_Ref,MOTION_INFO.Veh_Vx_Ref,MOTION_INFO.Veh_Vy_Ref,MOTION_INFO.Veh_AVy_Ref
  MATLAB Function : MATLAB Function  TreatAsAtomicUnit=on
  Mux : Mux  Inputs=2
  Scope : Scope  NumInputPorts=4
  Scope1 : Scope
  Scope2 : Scope
  Path_Error_Info : Outport
  wires:
  State/1 -> Bus Selector/1
  1-D Lookup Table/1 -> Mux/1, [Path_Theta_Est]
  1-D Lookup Table1/1 -> Mux/2, [Path_Kappa_Est]
  [Path_Theta_Est] -> MATLAB Function/1(Path_Theta_Est)
  [Path_Kappa_Est] -> MATLAB Function/2(Path_Kappa_Est)
  MATLAB Function/4(Veh_ErrAVz_Est) -> Scope/4, Bus Creator/4
  MATLAB Function/3(Veh_ErrYz_Est) -> Scope/3, Bus Creator/3
  MATLAB Function/2(Veh_ErrVy_Est) -> Scope/2, Bus Creator/2
  MATLAB Function/1(Veh_ErrY_Est) -> Scope/1, Bus Creator/1
  Bus Creator/1 -> Path_Error_Info/1  "PATH_ERROR_INFO"
  Mux/1 -> Scope2/1
  Bus Selector/1 -> [Path_S_Ref]  "<Path_S_Ref>"
  Bus Selector/2 -> [Path_L_Ref]  "<Path_L_Ref>"
  Bus Selector/3 -> Scope1/1, [Veh_Yz_Ref]  "<Veh_Yz_Ref>"
  Bus Selector/4 -> [Veh_Vx_Ref]  "<Veh_Vx_Ref>"
  Bus Selector/5 -> [Veh_Vy_Ref]  "<Veh_Vy_Ref>"
  Bus Selector/6 -> [Veh_AVy_Ref]  "<Veh_AVy_Ref>"
  [Path_S_Ref] -> 1-D Lookup Table/1, 1-D Lookup Table1/1
  [Path_L_Ref] -> MATLAB Function/3(Path_L_Ref)
  [Veh_Yz_Ref] -> MATLAB Function/4(Veh_Yz_Ref)
  [Veh_Vx_Ref] -> MATLAB Function/5(Veh_Vx_Ref)
  [Veh_Vy_Ref] -> MATLAB Function/6(Veh_Vy_Ref)
  [Veh_AVy_Ref] -> MATLAB Function/7(Veh_AVz_Ref)

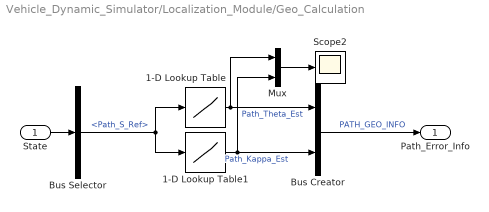
== system Vehicle_Dynamic_Simulator/Localization_Module/Geo_Calculation ==
  State : Inport
  1-D Lookup Table : Lookup_n-D  NumberOfTableDimensions=1  BreakpointsForDimension1=Path.S  Table=Path.Theta  InternalRulePriority=Speed  RndMeth=Simplest  InputSameDT=on
  1-D Lookup Table1 : Lookup_n-D  NumberOfTableDimensions=1  BreakpointsForDimension1=Path.S  Table=Path.Kappa  InternalRulePriority=Speed  RndMeth=Simplest  InputSameDT=on
  Bus Creator : BusCreator  Inputs=2
  Bus Selector : BusSelector  OutputSignals=PATH_INFO.Path_S_Ref
  Mux : Mux  Inputs=2
  Scope2 : Scope
  Path_Error_Info : Outport
  wires:
  Bus Selector/1 -> 1-D Lookup Table1/1, 1-D Lookup Table/1  "<Path_S_Ref>"
  Mux/1 -> Scope2/1
  Bus Creator/1 -> Path_Error_Info/1  "PATH_GEO_INFO"
  1-D Lookup Table1/1 -> Bus Creator/2, Mux/2  "Path_Kappa_Est"
  1-D Lookup Table/1 -> Bus Creator/1, Mux/1  "Path_Theta_Est"
  State/1 -> Bus Selector/1

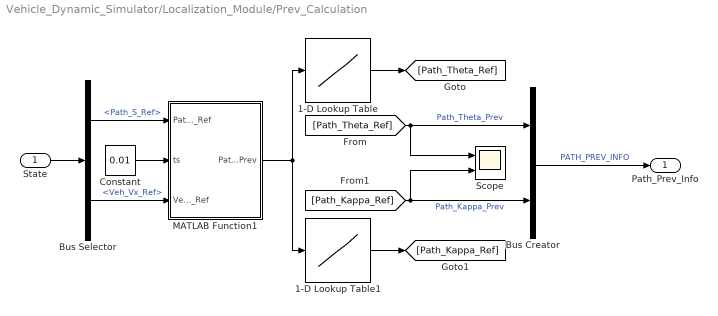
== system Vehicle_Dynamic_Simulator/Localization_Module/Prev_Calculation ==
  State : Inport
  1-D Lookup Table : Lookup_n-D  NumberOfTableDimensions=1  BreakpointsForDimension1=Path.S  Table=Path.Theta  InternalRulePriority=Speed  RndMeth=Simplest  InputSameDT=on
  1-D Lookup Table1 : Lookup_n-D  NumberOfTableDimensions=1  BreakpointsForDimension1=Path.S  Table=Path.Kappa  InternalRulePriority=Speed  RndMeth=Simplest  InputSameDT=on
  Bus Creator : BusCreator  Inputs=2
  Bus Selector : BusSelector  OutputSignals=PATH_INFO.Path_S_Ref,MOTION_INFO.Veh_Vx_Ref
  Constant : Constant  Value=0.01
  MATLAB Function1 : MATLAB Function  TreatAsAtomicUnit=on
  Scope : Scope  NumInputPorts=2
  Path_Prev_Info : Outport
  wires:
  State/1 -> Bus Selector/1
  1-D Lookup Table/1 -> [Path_Theta_Ref]
  1-D Lookup Table1/1 -> [Path_Kappa_Ref]
  Bus Selector/2 -> MATLAB Function1/3(Veh_Vx_Ref)  "<Veh_Vx_Ref>"
  Bus Selector/1 -> MATLAB Function1/1(Path_S_Ref)  "<Path_S_Ref>"
  MATLAB Function1/1(Path_S_Prev) -> 1-D Lookup Table/1, 1-D Lookup Table1/1
  [Path_Theta_Ref] -> Bus Creator/1, Scope/1  "Path_Theta_Prev"
  [Path_Kappa_Ref] -> Bus Creator/2, Scope/2  "Path_Kappa_Prev"
  Bus Creator/1 -> Path_Prev_Info/1  "PATH_PREV_INFO"
  Constant/1 -> MATLAB Function1/2(ts)

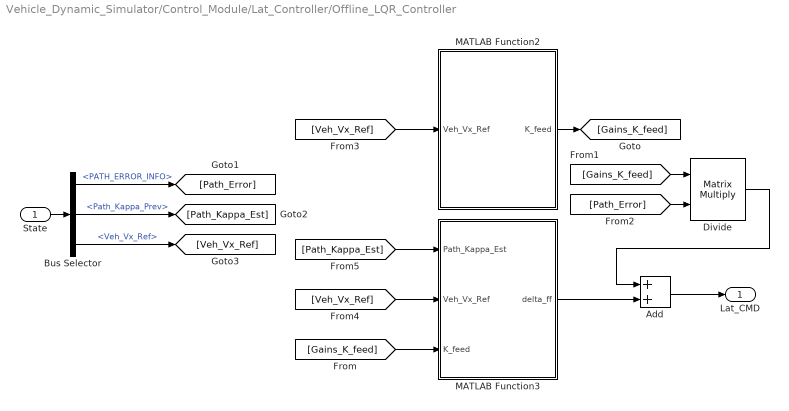
== system Vehicle_Dynamic_Simulator/Control_Module/Lat_Controller/Offline_LQR_Controller ==
  State : Inport
  Add : Sum
  Bus Selector : BusSelector  OutputSignals=LOCALIZATION_INFO.PATH_ERROR_INFO,LOCALIZATION_INFO.PATH_PREV_INFO.Path_Kappa_Prev,MOTION_INFO.Veh_Vx_Ref
  Divide : Product  Inputs=**  Multiplication=Matrix(*)
  MATLAB Function2 : MATLAB Function  TreatAsAtomicUnit=on
  MATLAB Function3 : MATLAB Function  TreatAsAtomicUnit=on
  Lat_CMD : Outport
  wires:
  State/1 -> Bus Selector/1
  MATLAB Function2/1(K_feed) -> [Gains_K_feed]
  [Gains_K_feed] -> MATLAB Function3/3(K_feed)
  Divide/1 -> Add/1
  MATLAB Function3/1(delta_ff) -> Add/2
  Bus Selector/1 -> [Path_Error]  "<PATH_ERROR_INFO>"
  Bus Selector/2 -> [Path_Kappa_Est]  "<Path_Kappa_Prev>"
  Bus Selector/3 -> [Veh_Vx_Ref]  "<Veh_Vx_Ref>"
  [Veh_Vx_Ref] -> MATLAB Function2/1(Veh_Vx_Ref)
  [Veh_Vx_Ref] -> MATLAB Function3/2(Veh_Vx_Ref)
  [Path_Kappa_Est] -> MATLAB Function3/1(Path_Kappa_Est)
  [Gains_K_feed] -> Divide/1
  [Path_Error] -> Divide/2
  Add/1 -> Lat_CMD/1

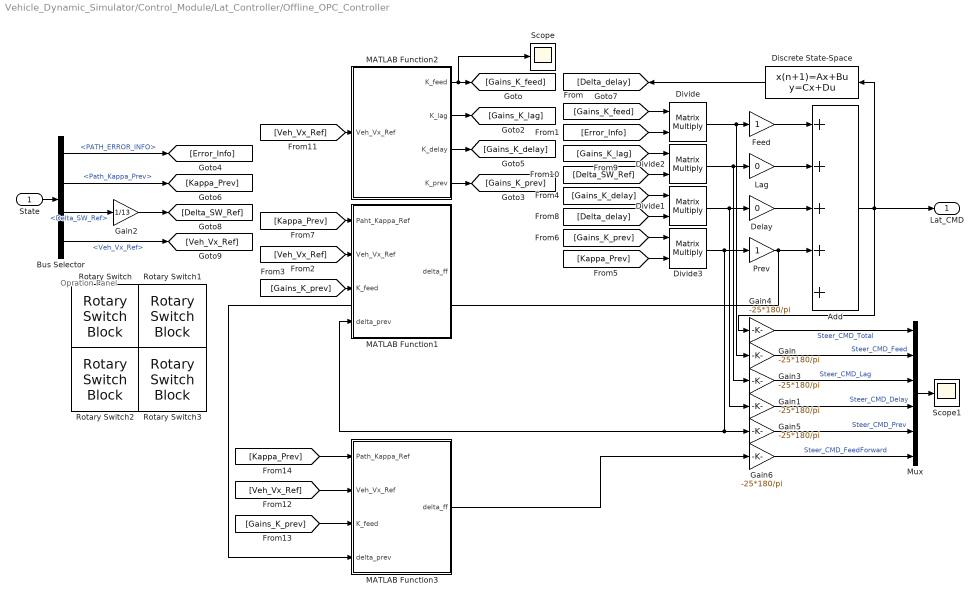
== system Vehicle_Dynamic_Simulator/Control_Module/Lat_Controller/Offline_OPC_Controller ==
  note: Opration Panel
  State : Inport
  Add : Sum  Inputs=+++++
  Bus Selector : BusSelector  OutputSignals=LOCALIZATION_INFO.PATH_ERROR_INFO,LOCALIZATION_INFO.PATH_PREV_INFO.Path_Kappa_Prev,MOTION_INFO.Delta_SW_Ref,MOTION_INFO.Veh_Vx_Ref
  Delay : Gain  Gain=0
  Discrete State-Space : DiscreteStateSpace  A=[zeros(19,1),eye(19);0,zeros(1,19)]  B=[zeros(19,1);1]  C=eye(20)  D=zeros(20,1)  InitialCondition=zeros(20,1)  SampleTime=-1
  Divide{,1..3} (4 alike) : Product  Inputs=**  Multiplication=Matrix(*)
  Feed : Gain
  Gain{,1,3..6} (6 alike) : Gain  Gain=-25*180/pi
  Gain2 : Gain  Gain=1/13
  Lag : Gain  Gain=0
  MATLAB Function1 : MATLAB Function  TreatAsAtomicUnit=on
  MATLAB Function2 : MATLAB Function  TreatAsAtomicUnit=on
  MATLAB Function3 : MATLAB Function  TreatAsAtomicUnit=on
  Mux : Mux  Inputs=6
  Prev : Gain
  Rotary Switch{,1..3} (4 alike) : RotarySwitchBlock
      settings: Values={{'Off', 'Low', 'Medium', 'High', 'Full'}, [0 0.25 0.5 0.75 1]}
  Scope : Scope
  Scope1 : Scope
  Lat_CMD : Outport
  wires:
  State/1 -> Bus Selector/1
  MATLAB Function2/1(K_feed) -> Scope/1, [Gains_K_feed]
  [Gains_K_feed] -> Divide/1
  [Error_Info] -> Divide/2
  [Gains_K_prev] -> Divide3/1
  [Kappa_Prev] -> Divide3/2
  Divide/1 -> Feed/1, Gain/1
  Mux/1 -> Scope1/1
  Bus Selector/1 -> [Error_Info]  "<PATH_ERROR_INFO>"
  Bus Selector/2 -> [Kappa_Prev]  "<Path_Kappa_Prev>"
  Add/1 -> Discrete State-Space/1, Gain4/1, Lat_CMD/1
  [Kappa_Prev] -> MATLAB Function1/1(Paht_Kappa_Ref)
  [Gains_K_prev] -> MATLAB Function1/3(K_feed)
  Divide3/1 -> Prev/1, MATLAB Function1/4(delta_prev), Gain5/1
  MATLAB Function2/2(K_lag) -> [Gains_K_lag]
  MATLAB Function2/3(K_delay) -> [Gains_K_delay]
  [Gains_K_delay] -> Divide1/1
  [Gains_K_lag] -> Divide2/1
  Divide2/1 -> Lag/1, Gain3/1
  Divide1/1 -> Delay/1, Gain1/1
  [Delta_SW_Ref] -> Divide2/2
  [Delta_delay] -> Divide1/2
  MATLAB Function2/4(K_prev) -> [Gains_K_prev]
  Discrete State-Space/1 -> [Delta_delay]
  Gain5/1 -> Mux/5  "Steer_CMD_Prev"
  Gain1/1 -> Mux/4  "Steer_CMD_Delay"
  Gain3/1 -> Mux/3  "Steer_CMD_Lag"
  Gain/1 -> Mux/2  "Steer_CMD_Feed"
  Gain4/1 -> Mux/1  "Steer_CMD_Total"
  Feed/1 -> Add/1
  Lag/1 -> Add/2
  Delay/1 -> Add/3
  Prev/1 -> Add/4, MATLAB Function3/4(delta_prev)
  Gain6/1 -> Mux/6  "Steer_CMD_FeedForward"
  [Veh_Vx_Ref] -> MATLAB Function1/2(Veh_Vx_Ref)
  [Veh_Vx_Ref] -> MATLAB Function2/1(Veh_Vx_Ref)
  Bus Selector/3 -> Gain2/1  "<Delta_SW_Ref>"
  Bus Selector/4 -> [Veh_Vx_Ref]  "<Veh_Vx_Ref>"
  Gain2/1 -> [Delta_SW_Ref]
  [Kappa_Prev] -> MATLAB Function3/1(Path_Kappa_Ref)
  [Veh_Vx_Ref] -> MATLAB Function3/2(Veh_Vx_Ref)
  [Gains_K_prev] -> MATLAB Function3/3(K_feed)
  MATLAB Function3/1(delta_ff) -> Gain6/1

== system Vehicle_Dynamic_Simulator/Control_Module/Lat_Controller/Online_MPC_Controller ==
  State : Inport
  MPC Controller : mpclib/MPC Controller  SCDEnableBlockLinearizationSpecification=on  mpcobj=Lateral_MPC  is_multiple=0  enable_value=0  return_u0=off  updateMPCinCallerWorkspace=on  md_inport=on  mv_inport=off  uref_inport=off  return_cost=off  return_mvseq=off  return_qpstatus=off  return_xseq=off  return_state=off  return_ovseq=off  state_inport=off  umin_inport=off  umax_inport=off  ymin_inport=off  ymax_inport=off  cc_inport=off  ywt_inport=off  uwt_inport=off  duwt_inport=off  rhoeps_inport=off  pm_inport=off  MaximumP=10  HorizonChoice=FixedHorizon  n_ts=1  n_p=10  n_mv=1  n_md=1  n_ud=0  n_mo=1  n_uo=0  BlockDataType=double  SampleTimeInherited=off  switch_inport=off
  Lat_CMD : Outport
  wires:
  State/1 -> ?
  MPC Controller/1 -> Lat_CMD/1

== system Vehicle_Dynamic_Simulator/Control_Module/Lat_Controller/Stanley_Controller ==
  State : Inport
  Bus Selector : BusSelector  OutputSignals=LOCALIZATION_INFO.PATH_ERROR_INFO.Veh_ErrY_Est,LOCALIZATION_INFO.PATH_ERROR_INFO.Veh_ErrYz_Est,MOTION_INFO.Veh_Vx_Ref,MOTION_INFO.Veh_Vy_Ref,MOTION_INFO.Veh_AVz_Ref,MOTION_INFO.Delta_SW_Ref
  MATLAB Function1 : MATLAB Function  TreatAsAtomicUnit=on
  MATLAB Function2 : MATLAB Function  TreatAsAtomicUnit=on
  Lat_CMD : Outport
  wires:
  State/1 -> Bus Selector/1
  Bus Selector/3 -> MATLAB Function2/1(Veh_Vx_Ref), MATLAB Function1/3(vx_veh_ref)  "<Veh_Vx_Ref>"
  Bus Selector/2 -> MATLAB Function1/2(error_phi)  "<Veh_ErrYz_Est>"
  Bus Selector/1 -> MATLAB Function1/1(error_y)  "<Veh_ErrY_Est>"
  MATLAB Function1/1(Lat_CMD) -> Lat_CMD/1  "Lat_CMD"
  Bus Selector/4 -> MATLAB Function1/4(vy_veh_ref)  "<Veh_Vy_Ref>"
  Bus Selector/5 -> MATLAB Function1/5(avz_veh_ref)  "<Veh_AVz_Ref>"
  Bus Selector/6 -> MATLAB Function1/6(delta_sw)  "<Delta_SW_Ref>"
  MATLAB Function2/1(K_feed) -> MATLAB Function1/7(gain)

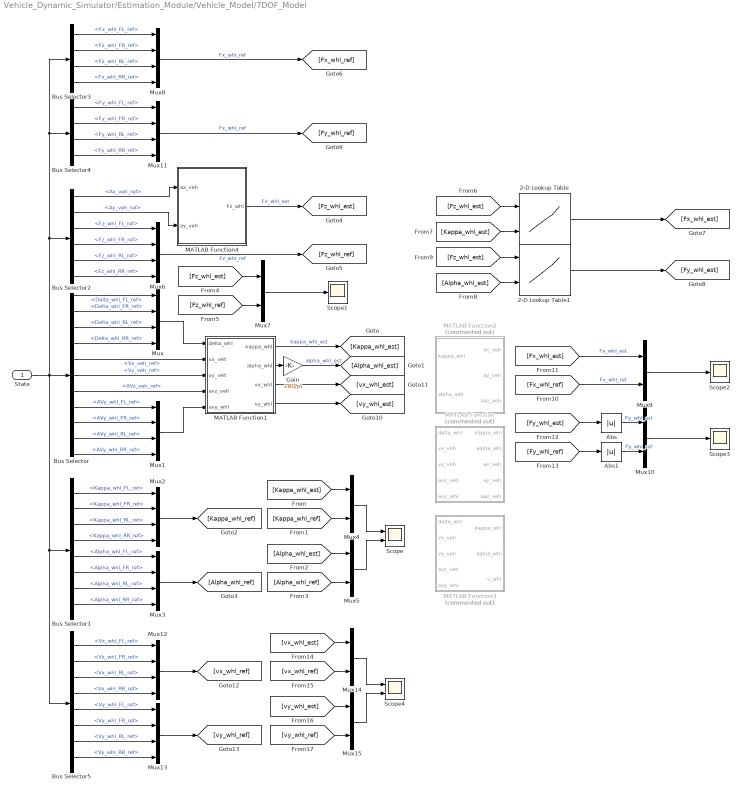
== system Vehicle_Dynamic_Simulator/Estimation_Module/Vehicle_Model/7DOF_Model ==
  State : Inport
  2-D Lookup Table : Lookup_n-D  BreakpointsForDimension1=Fz  BreakpointsForDimension2=Kappa  Table=Fx'  InternalRulePriority=Speed  RndMeth=Simplest  InputSameDT=on
      settings: InputPortMap=u0,u1
  2-D Lookup Table1 : Lookup_n-D  BreakpointsForDimension1=Fz  BreakpointsForDimension2=Alpha  Table=Fy'  InternalRulePriority=Speed  RndMeth=Simplest  InputSameDT=on
      settings: InputPortMap=u0,u1
  Abs : Abs
  Abs1 : Abs
  Bus Selector : BusSelector  OutputSignals=Chassis_Info.Delta_whl_FL_ref,Chassis_Info.Delta_whl_FR_ref,Chassis_Info.Delta_whl_RL_ref,Chassis_Info.Delta_whl_RR_ref,Chassis_Info.Vx_veh_ref,Chassis_Info.Vy_veh_ref,Chassis_Info.AVz_veh_ref,Chassis_Info.AVy_whl_FL_ref,Chassis_Info.AVy_whl_FR_ref,Chassis_Info.AVy_whl_RL_ref,Chassis_Info.AVy_whl_RR_ref
  Bus Selector1 : BusSelector  OutputSignals=Chassis_Info.Kappa_whl_FL_ref,Chassis_Info.Kappa_whl_FR_ref,Chassis_Info.Kappa_whl_RL_ref,Chassis_Info.Kappa_whl_RR_ref,Chassis_Info.Alpha_whl_FL_ref,Chassis_Info.Alpha_whl_FR_ref,Chassis_Info.Alpha_whl_RL_ref,Chassis_Info.Alpha_whl_RR_ref
  Bus Selector2 : BusSelector  OutputSignals=Chassis_Info.Ax_veh_ref,Chassis_Info.Ay_veh_ref,Chassis_Info.Fz_whl_FL_ref,Chassis_Info.Fz_whl_FR_ref,Chassis_Info.Fz_whl_RL_ref,Chassis_Info.Fz_whl_RR_ref
  Bus Selector3 : BusSelector  OutputSignals=Chassis_Info.Fx_whl_FL_ref,Chassis_Info.Fx_whl_FR_ref,Chassis_Info.Fx_whl_RL_ref,Chassis_Info.Fx_whl_RR_ref
  Bus Selector4 : BusSelector  OutputSignals=Chassis_Info.Fy_whl_FL_ref,Chassis_Info.Fy_whl_FR_ref,Chassis_Info.Fy_whl_RL_ref,Chassis_Info.Fy_whl_RR_ref
  Bus Selector5 : BusSelector  OutputSignals=Chassis_Info.Vx_whl_FL_ref,Chassis_Info.Vx_whl_FR_ref,Chassis_Info.Vx_whl_RL_ref,Chassis_Info.Vx_whl_RR_ref,Chassis_Info.Vy_whl_FL_ref,Chassis_Info.Vy_whl_FR_ref,Chassis_Info.Vy_whl_RL_ref,Chassis_Info.Vy_whl_RR_ref
  Gain : Gain  Gain=180/pi
  MATLAB Function : MATLAB Function  Commented=on  TreatAsAtomicUnit=on
  MATLAB Function1 : MATLAB Function  TreatAsAtomicUnit=on
  MATLAB Function2 : MATLAB Function  Commented=on  TreatAsAtomicUnit=on
  MATLAB Function3 : MATLAB Function  Commented=on  TreatAsAtomicUnit=on
  MATLAB Function4 : MATLAB Function  TreatAsAtomicUnit=on
  Mux{,1..3,6,8,11..13} (9 alike) : Mux
  Mux{4..5,7,9..10,14..15} (7 alike) : Mux  Inputs=2
  Scope : Scope  NumInputPorts=2
  Scope1 : Scope
  Scope2 : Scope
  Scope3 : Scope
  Scope4 : Scope  NumInputPorts=2
  wires:
  State/1 -> Bus Selector2/1, Bus Selector3/1, Bus Selector4/1, Bus Selector1/1, Bus Selector5/1, Bus Selector/1
  Bus Selector/5 -> MATLAB Function1/2(vx_veh)  "<Vx_veh_ref>"
  Bus Selector/6 -> MATLAB Function1/3(vy_veh)  "<Vy_veh_ref>"
  Bus Selector/7 -> MATLAB Function1/4(avz_veh)  "<AVz_veh_ref>"
  Bus Selector/4 -> Mux/4  "<Delta_whl_RR_ref>"
  Bus Selector/3 -> Mux/3  "<Delta_whl_RL_ref>"
  Bus Selector/2 -> Mux/2  "<Delta_whl_FR_ref>"
  Bus Selector/1 -> Mux/1  "<Delta_whl_FL_ref>"
  Mux/1 -> MATLAB Function1/1(delta_whl)
  Bus Selector/8 -> Mux1/1  "<AVy_whl_FL_ref>"
  Bus Selector/9 -> Mux1/2  "<AVy_whl_FR_ref>"
  Bus Selector/10 -> Mux1/3  "<AVy_whl_RL_ref>"
  Bus Selector/11 -> Mux1/4  "<AVy_whl_RR_ref>"
  Mux1/1 -> MATLAB Function1/5(avy_whl)
  MATLAB Function1/1(kappa_whl) -> [Kappa_whl_est]  "kappa_whl_est"
  MATLAB Function1/2(alpha_whl) -> Gain/1
  Gain/1 -> [Alpha_whl_est]  "alpha_whl_est"
  Bus Selector1/1 -> Mux2/1  "<Kappa_whl_FL_ref>"
  Bus Selector1/2 -> Mux2/2  "<Kappa_whl_FR_ref>"
  Bus Selector1/3 -> Mux2/3  "<Kappa_whl_RL_ref>"
  Bus Selector1/4 -> Mux2/4  "<Kappa_whl_RR_ref>"
  Bus Selector1/5 -> Mux3/1  "<Alpha_whl_FL_ref>"
  Bus Selector1/6 -> Mux3/2  "<Alpha_whl_FR_ref>"
  Bus Selector1/7 -> Mux3/3  "<Alpha_whl_RL_ref>"
  Bus Selector1/8 -> Mux3/4  "<Alpha_whl_RR_ref>"
  Mux2/1 -> [Kappa_whl_ref]
  Mux3/1 -> [Alpha_whl_ref]
  [Kappa_whl_ref] -> Mux4/2
  [Kappa_whl_est] -> Mux4/1
  [Alpha_whl_est] -> Mux5/1
  [Alpha_whl_ref] -> Mux5/2
  Mux4/1 -> Scope/1
  Mux5/1 -> Scope/2
  Bus Selector2/2 -> MATLAB Function4/2(ay_veh)  "<Ay_veh_ref>"
  Bus Selector2/1 -> MATLAB Function4/1(ax_veh)  "<Ax_veh_ref>"
  Bus Selector2/6 -> Mux6/4  "<Fz_whl_RR_ref>"
  Bus Selector2/5 -> Mux6/3  "<Fz_whl_RL_ref>"
  Bus Selector2/4 -> Mux6/2  "<Fz_whl_FR_ref>"
  Bus Selector2/3 -> Mux6/1  "<Fz_whl_FL_ref>"
  MATLAB Function4/1(Fz_whl) -> [Fz_whl_est]  "Fz_whl_est"
  Mux6/1 -> [Fz_whl_ref]  "Fz_whl_ref"
  [Fz_whl_est] -> Mux7/1
  [Fz_whl_ref] -> Mux7/2
  Mux7/1 -> Scope1/1
  [Fz_whl_est] -> 2-D Lookup Table/1
  [Kappa_whl_est] -> 2-D Lookup Table/2
  [Fz_whl_est] -> 2-D Lookup Table1/1
  [Alpha_whl_est] -> 2-D Lookup Table1/2
  Bus Selector3/1 -> Mux8/1  "<Fx_whl_FL_ref>"
  Bus Selector3/2 -> Mux8/2  "<Fx_whl_FR_ref>"
  Bus Selector3/3 -> Mux8/3  "<Fx_whl_RL_ref>"
  Bus Selector3/4 -> Mux8/4  "<Fx_whl_RR_ref>"
  Mux8/1 -> [Fx_whl_ref]  "Fx_whl_ref"
  Mux9/1 -> Scope2/1
  [Fx_whl_ref] -> Mux9/2  "Fx_whl_ref"
  [Fx_whl_est] -> Mux9/1  "Fx_whl_est"
  Mux10/1 -> Scope3/1
  Bus Selector4/1 -> Mux11/1  "<Fy_whl_FL_ref>"
  Bus Selector4/2 -> Mux11/2  "<Fy_whl_FR_ref>"
  Bus Selector4/3 -> Mux11/3  "<Fy_whl_RL_ref>"
  Bus Selector4/4 -> Mux11/4  "<Fy_whl_RR_ref>"
  Mux11/1 -> [Fy_whl_ref]  "Fx_whl_ref"
  [Fy_whl_ref] -> Abs1/1
  Abs1/1 -> Mux10/2  "Fy_whl_ref"
  [Fy_whl_est] -> Abs/1
  Abs/1 -> Mux10/1  "Fy_whl_est"
  2-D Lookup Table/1 -> [Fx_whl_est]
  2-D Lookup Table1/1 -> [Fy_whl_est]
  MATLAB Function1/4(vy_whl) -> [vy_whl_est]
  MATLAB Function1/3(vx_whl) -> [vx_whl_est]
  Bus Selector5/1 -> Mux12/1  "<Vx_whl_FL_ref>"
  Bus Selector5/2 -> Mux12/2  "<Vx_whl_FR_ref>"
  Bus Selector5/3 -> Mux12/3  "<Vx_whl_RL_ref>"
  Bus Selector5/4 -> Mux12/4  "<Vx_whl_RR_ref>"
  Bus Selector5/5 -> Mux13/1  "<Vy_whl_FL_ref>"
  Bus Selector5/6 -> Mux13/2  "<Vy_whl_FR_ref>"
  Bus Selector5/7 -> Mux13/3  "<Vy_whl_RL_ref>"
  Bus Selector5/8 -> Mux13/4  "<Vy_whl_RR_ref>"
  Mux12/1 -> [vx_whl_ref]
  Mux13/1 -> [vy_whl_ref]
  [vx_whl_est] -> Mux14/1
  [vx_whl_ref] -> Mux14/2
  [vy_whl_ref] -> Mux15/2
  [vy_whl_est] -> Mux15/1
  Mux15/1 -> Scope4/2
  Mux14/1 -> Scope4/1

== matlab function Vehicle_Dynamic_Simulator/Estimation_Module/Vehicle_Model/7DOF_Model/MATLAB Function1 ==
  data: delta_whl input; kappa_whl output; vx_veh input; vy_veh input; avz_veh input; alpha_whl output; avy_whl input; vx_whl output; vy_whl output
function [kappa_whl, alpha_whl, vx_whl, vy_whl] = ...
    Compute_Tyre_Kinematics(delta_whl, vx_veh, vy_veh, avz_veh, avy_whl)
% Vehicle Parameters
     L  = [+1.265; +1.265; -1.895; -1.895];
     W  = [+0.802; -0.802; +0.802; -0.802];    
         
     R_whl = 0.368;
% Calculate Tyre Kinematic
    vx_whl = zeros(4,1);
    vy_whl = zeros(4,1);
     v_whl = zeros(4,1);

    kappa_whl = zeros(4,1);
    alpha_whl = zeros(4,1);

    for i = 1:1:4
        vx_whl(i,1) = + vx_veh - W(i,1)*avz_veh;
        vy_whl(i,1) = + vy_veh + L(i,1)*avz_veh;
         v_whl(i,1) = cos(delta_whl(i,1))*sqrt(vx_whl(i,1)^2 + vy_whl(i,1)^2);

        kappa_whl(i,1) = (avy_whl(i,1)*R_whl - v_whl(i,1))/v_whl(i,1); 
        alpha_whl(i,1) = atan(vy_whl(i,1)/vx_whl(i,1)) - delta_whl(i,1);
    end
end

== matlab function Vehicle_Dynamic_Simulator/Estimation_Module/Vehicle_Model/7DOF_Model/MATLAB Function2 ==
  data: kappa_whl input; alpha_whl input; ax_veh output; ay_veh output; aaz_veh output
function [ax_veh, ay_veh, aaz_veh] = ...
    Vehicle_Model(kappa_whl, alpha_whl)
% Vehicle Parameters
     W  = [+0.775; -0.775; +0.825; -0.825];    
     L  = [+0.970; +0.970; -1.810; -1.810];
     Kx = [+45000; +45000; +45000; +45000];      
     Ky = [-50000; -50000; -50000; -50000];    
     M  = 1521;                  
     Iz = 1816;          

% Calculate State   
     ax_veh =  vy_veh*avz_veh;
     ay_veh = -vx_veh*avz_veh;
    aaz_veh = 0;
    for i = 1:1:4
        ax_veh = ax_veh + ...
            (1/M)*(Kx(i,1)*kappa_whl(i,1)*cos(delta_whl(i,1)) - ...
                   Ky(i,1)*alpha_whl(i,1)*sin(delta_whl(i,1)));
        ay_veh = ay_veh + ...
            (1/M)*(Kx(i,1)*kappa_whl(i,1)*sin(delta_whl(i,1)) + ...
                   Ky(i,1)*alpha_whl(i,1)*cos(delta_whl(i,1)));
        aaz_veh = aaz_veh + ...
            (1/Iz)*(-W(i,1))*...
            (Kx(i,1)*kappa_whl(i,1)*cos(delta_whl(i,1)) - ...
             Ky(i,1)*alpha_whl(i,1)*sin(delta_whl(i,1))) + ...
            (1/Iz)*(L(i,1))*...
            (Kx(i,1)*kappa_whl(i,1)*sin(delta_whl(i,1)) - ...
             Ky(i,1)*alpha_whl(i,1)*cos(delta_whl(i,1)));
    end
end

== matlab function Vehicle_Dynamic_Simulator/Control_Module/Lat_Controller/Stanley_Controller/MATLAB Function1 ==
  data: Lat_CMD output; error_y input; error_phi input; vx_veh_ref input; vy_veh_ref input; avz_veh_ref input; delta_sw input; gain input
function Lat_CMD = Compute_Stanley(error_y, error_phi, vx_veh_ref, vy_veh_ref, avz_veh_ref, delta_sw, gain)
    vf = vx_veh_ref + 0.04*(vy_veh_ref + 1.265*avz_veh_ref)*delta_sw;
    Lat_CMD = error_phi + atan((gain*error_y)/(vf + 0.01));
end

== matlab function Vehicle_Dynamic_Simulator/Control_Module/Lat_Controller/Offline_OPC_Controller/MATLAB Function1 ==
  data: delta_ff output; Paht_Kappa_Ref input; Veh_Vx_Ref input; K_feed input; delta_prev input
function delta_ff   = OPC_FeedForward(Paht_Kappa_Ref, Veh_Vx_Ref, K_feed, delta_prev)
    MT = 2020; IZ = 4095; LF = 1.265; LR = 1.895; KF = -70000; KR = -70000;
    
    a23 = -2*(KF+KR)/MT;
    a43 = -2*(KF*LF-KR*LR)/IZ;	
	b21 = -2*KF/MT;

    b41 = -2*KF*LF/IZ;
	d21 = 2*(KF*LF-KR*LR)/MT - Veh_Vx_Ref*Veh_Vx_Ref;		
    d41 = 2*(KF*LF*LF+KR*LR*LR)/IZ;


    k1 = K_feed(1,1);
    k3 = K_feed(1,3);

    Paht_Kappa_Ref = Paht_Kappa_Ref(1,1);
    delta_ff = (((b21*delta_prev - d21*Paht_Kappa_Ref)*(a43 - b41*k3))/(a23*b41*k1 - a43*b21*k1) - ((b41*delta_prev - d41*Paht_Kappa_Ref)*(a23 - b21*k3))/(a23*b41*k1 - a43*b21*k1))/((b41*(a23 - b21*k3))/(a23*b41*k1 - a43*b21*k1) - (b21*(a43 - b41*k3))/(a23*b41*k1 - a43*b21*k1));
end

== matlab function Vehicle_Dynamic_Simulator/Control_Module/Lat_Controller/Offline_OPC_Controller/MATLAB Function3 ==
  data: delta_ff output; Path_Kappa_Ref input; Veh_Vx_Ref input; K_feed input; delta_prev input
function delta_ff   = OPC_FeedForward(Path_Kappa_Ref, Veh_Vx_Ref, K_feed, delta_prev)
    MT = 2020; IZ = 4095; LF = 1.265; LR = 1.895; KF = -70000; KR = -70000;
    Path_Kappa_Ref = Path_Kappa_Ref(1,1);
    a23 = -2*(KF+KR)/MT;
    a43 = -2*(KF*LF-KR*LR)/IZ;	
	b21 = -2*KF/MT;

    b41 = -2*KF*LF/IZ;
	d21 = 2*(KF*LF-KR*LR)/MT - Veh_Vx_Ref*Veh_Vx_Ref;		
    d41 = 2*(KF*LF*LF+KR*LR*LR)/IZ;

    k1 = K_feed(1,1);
    k3 = K_feed(1,3);
    A = a23 - k3*b21;
    B = a43 - k3*b41;

    delta_ff = - delta_prev - ((A*d41 - B*d21)/(A*b41 - B*b21))*Path_Kappa_Ref;
end

== matlab function Vehicle_Dynamic_Simulator/Control_Module/Lat_Controller/Offline_LQR_Controller/MATLAB Function2 ==
  data: K_feed output; Veh_Vx_Ref input
function K_feed  = LQR_K_Interpolation(Veh_Vx_Ref)
    K_table = load("Controllers\Lateral_Controller\Optimal_Preview_Controller\Conf\optimal_preview_K_table.mat");
    K_table = K_table.OPC_K_Table;
    
    K_feed = zeros(1,4);

    for i=1:1:4
        K_feed(1,i) = interp1(K_table(:,2), K_table(:,i+2), Veh_Vx_Ref, 'linear', 'extrap');
    end
end

== matlab function Vehicle_Dynamic_Simulator/MATLAB Function ==
  data: Time input; FLAG_Trigger output
function FLAG_Trigger = Trigger(Time)
    if mod(Time, 0.01) == 0
        FLAG_Trigger = 1;
    else
        FLAG_Trigger = 0;
    end
end

== matlab function Vehicle_Dynamic_Simulator/Control_Module/Lat-Lon Controller/MATLAB Function2 ==
  data: Veh_Beta_dot_Des output; Veh_ErrY input; Veh_AAz_Des output
function [Veh_Beta_dot_Des, Veh_AAz_Des]  = Imposed_Error_Dynamics(Veh_ErrY)
    Kp = 2.0;
    Kd = 2.8;
    Kb = 2.0;

    Veh_Beta_dot_Des = (-);
    Veh_AAz_Des = ;
end

== matlab function Vehicle_Dynamic_Simulator/Estimation_Module/Vehicle_Model/7DOF_Model/MATLAB Function3 ==
  data: delta_whl input; kappa_whl output; vx_veh input; vy_veh input; avz_veh input; alpha_whl output; avy_whl input; v_whl output
function [kappa_whl, alpha_whl, v_whl] = ...
    Compute_Tyre_Dynamics(delta_whl, vx_veh, vy_veh, avz_veh, avy_whl)
% Vehicle Parameters
     W  = [+0.775; -0.775; +0.825; -0.825];    
     L  = [+0.970; +0.970; -1.810; -1.810];
    
     M  = 1521;                  
     Iz = 1816;          
     R_whl = 0.329;
% Calculate Tyre Kinematic
    vx_whl = zeros(4,1);
    vy_whl = zeros(4,1);
     v_whl = zeros(4,1);

    kappa_whl = zeros(4,1);
    alpha_whl = zeros(4,1);

    for i = 1:1:4
        vx_whl(i,1) = vx_veh - W(i,1)*avz_veh;
        vy_whl(i,1) = vy_veh + L(i,1)*avz_veh;
         v_whl(i,1) = cos(delta_whl(i,1))*sqrt(vx_whl(i,1)^2 + vy_whl(i,1)^2);

        kappa_whl(i,1) = (avy_whl(i,1)*R_whl - v_whl(i,1))/v_whl(i,1); 
        alpha_whl(i,1) = atan(vy_whl(i,1)/vx_whl(i,1)) - delta_whl(i,1);
    end
end

== matlab function Vehicle_Dynamic_Simulator/Estimation_Module/Vehicle_Model/7DOF_Model/MATLAB Function4 ==
  data: ax_veh input; Fz_whl output; ay_veh input
function Fz_whl  = ...
    Compute_Tyre_Dynamics(ax_veh, ay_veh)
% Vehicle Parameters
    M =  2020;
    H  = 0.39;
% Calculate Tyre Kinematic
    Fz_whl = [5841; 5841; 4062; 4062];
    coeffa = [-1; -1; +1; +1];
    coeffb = [-1.895; 1.895; -1.265; +1.265];
    for i = 1:1:4
        Fz_whl(i,1) = Fz_whl(i,1) + ax_veh*coeffa(i,1)*M*H/(2*3.16) + ...
                                    ay_veh*coeffb(i,1)*M*H/(1.605*3.16);
    end
end

== matlab function Vehicle_Dynamic_Simulator/Control_Module/Lat_Controller/Offline_LQR_Controller/MATLAB Function3 ==
  data: delta_ff output; Path_Kappa_Est input; Veh_Vx_Ref input; K_feed input
function delta_ff   = OPC_FeedForward(Path_Kappa_Est, Veh_Vx_Ref, K_feed)
    MT = 2020; IZ = 4095; LF = 1.265; LR = 1.895; KF = -70000; KR = -70000;
    Path_Kappa_Est = Path_Kappa_Est(1,1);
    a23 = -2*(KF+KR)/MT;
    a43 = -2*(KF*LF-KR*LR)/IZ;	
	b21 = -2*KF/MT;

    b41 = -2*KF*LF/IZ;
	d21 = 2*(KF*LF-KR*LR)/MT - Veh_Vx_Ref*Veh_Vx_Ref;		
    d41 = 2*(KF*LF*LF+KR*LR*LR)/IZ;

    k3 = K_feed(1,3);

    A = a23 - k3*b21;
    B = a43 - k3*b41;

    delta_ff = ((A*d41 - B*d21)/(A*b41 - B*b21))*Path_Kappa_Est;
end
